simulink model "condenser"  (R2018b)
settings: Solver=VariableStepAuto  StartTime=0.0  StopTime=10.0  RelTol=1e-3
settings Model: Creator=sofi  LastModifiedBy=art58

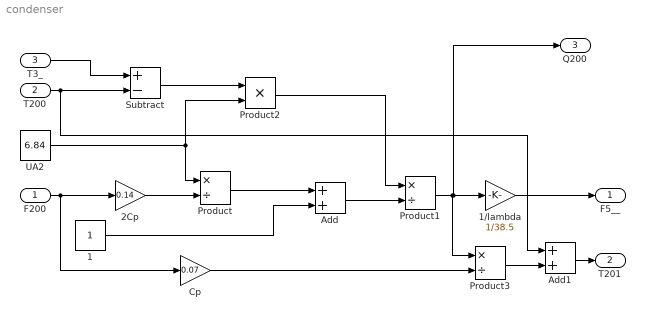
== system condenser ==
  F200 : Inport
  "T200 " : Inport  Port=2
  T3_ : Inport  Port=3
  1 : Constant
  1/lambda : Gain  Gain=1/38.5
  2Cp : Gain  Gain=0.14
  Add : Sum
  Add1 : Sum
  Cp : Gain  Gain=0.07
  Product : Product  Inputs=*/
  Product1 : Product  Inputs=*/
  Product2 : Product
  Product3 : Product  Inputs=*/
  Subtract : Sum  Inputs=+-
  UA2 : Constant  Value=6.84
  F5__ : Outport
  T201 : Outport  Port=2
  Q200 : Outport  Port=3
  wires:
  2Cp/1 -> Product/2
  UA2/1 -> Product/1, Product2/2
  Product/1 -> Add/1
  1/1 -> Add/2
  Add/1 -> Product1/2
  "T200 "/1 -> Add1/1, Subtract/2
  T3_/1 -> Subtract/1
  Subtract/1 -> Product2/1
  Product2/1 -> Product1/1
  Product1/1 -> Q200/1, 1/lambda/1, Product3/1
  1/lambda/1 -> F5__/1
  F200/1 -> Cp/1, 2Cp/1
  Cp/1 -> Product3/2
  Product3/1 -> Add1/2
  Add1/1 -> T201/1
